simulink model "block_vs_mfcn"  (Simulink 8.6)
settings: Solver=FixedStepDiscrete  SolverMode=SingleTasking  StartTime=0.0  StopTime=1e6  FixedStep=0.1  RelTol=1e-3
libraries: simulink x1
settings Model: Creator=gcampa  LastModifiedBy=gcampa
settings DataIOCC: LimitDataPoints=off  SaveFormat=Dataset  SignalLoggingSaveFormat=Dataset  ReturnWorkspaceOutputs=on
settings OptimizationCC: ExpressionDepthLimit=128
settings DebuggingCC: UnderspecifiedInitializationDetection=Simplified  MergeDetectMultiDrivingBlocksExec=error  SolverPrmCheckMsg=none  FcnCallInpInsideContextMsg=EnableAllAsError  AllowSymbolicDim=on  StateNameClashWarn=none  SFUnexpectedBacktrackingDiag=error  SFNoUnconditionalDefaultTransitionDiag=error
settings HardwareCC: ProdBitPerPointer=64  ProdLargestAtomicFloat=Float  ProdIntDivRoundTo=Zero  ProdEndianess=LittleEndian  ProdHWDeviceType=Specified
settings ModelReferenceCC: PropagateSignalLabelsOutOfModel=on
settings SFSimCC: SimUseLocalCustomCode=on
settings RTWCC: RTWUseLocalCustomCode=on
settings GRTTargetCC: TargetLangStandard=C99 (ISO)  CombineOutputUpdateFcns=on  GRTInterface=off
settings ConfigComp: CovMetricSettings=dwe  CovSaveCumulativeToWorkspaceVar=off  CovSaveSingleToWorkspaceVar=off  CovExternalEMLEnable=on

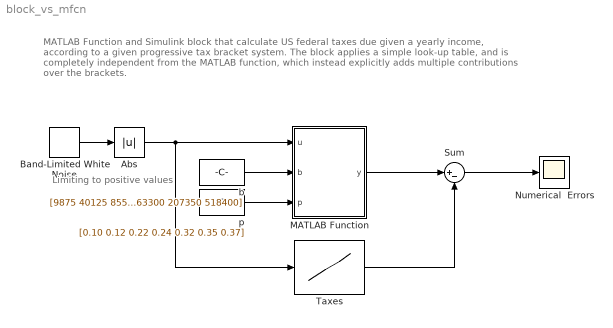
== system block_vs_mfcn ==
  note: MATLAB Function and Simulink block that calculate US federal taxes due given a yearly income, according to a given progressive tax bracket system.
      |
      | The block applies a simple look-up table, and is completely independent from the MATLAB function, which instead explicitly adds multiple contributions over the brackets.
  note: Limiting to
      | positive values
  Abs : Abs
  Band-Limited White Noise : simulink/Sources/Band-Limited White Noise  Cov=1e15  Ts=1  seed=[23341]
  MATLAB Function : MATLAB Function  TreatAsAtomicUnit=on
  Numerical  Errors : Scope
  Sum : Sum  Inputs=|+-
  Taxes : Lookup_n-D  NumberOfTableDimensions=1  BreakpointsForDimension1=xT  Table=yT  InternalRulePriority=Speed  RndMeth=Simplest  InputSameDT=on  mask(Taxes Look Up table){x=[9875 40125 85525 163300 207350 518400], p=[0.10 0.12 0.22 0.24 0.32 0.35 0.37]}
      mask prompts: x "Bracket upper limits"; p "Bracket tax rates"
      mask help:
      | This block calculates the taxes due for a given yearly income, according to a given progressive tax bracket system.
      | The input is the yearly income, the output is the tax amount due. The bracket upper limits and rates are the two mask parameter.
      | The first rate applies to income below the first upper limit and the last rate applies for incomes above the last upper limit.
      mask init:
      | xT=[0,x(:)',2*x(end)];
      | yT=0; for i=1:length(xT)-1, yT(i+1)=yT(i)+(xT(i+1)-xT(i))*p(i); end
  b : Constant  Value=[9875 40125 85525 163300 207350 518400]
  p : Constant  Value=[0.10 0.12 0.22 0.24 0.32 0.35 0.37]
  wires:
  Band-Limited White Noise/1 -> Abs/1
  b/1 -> MATLAB Function/2(b)
  p/1 -> MATLAB Function/3(p)
  MATLAB Function/1(y) -> Sum/1
  Taxes/1 -> Sum/2
  Sum/1 -> Numerical  Errors/1
  Abs/1 -> Taxes/1, MATLAB Function/1(u)

== matlab function MATLAB Function ==
  data: u input double; b input double; y output double; p input double
function y = fcn(u,b,p)

y=taxes(u,b,p);
